simulink model "BWQWFPIDKZhShChU"  (Simulink 5.0)
settings: Solver=ode45  StartTime=0.0  StopTime=200  FixedStep=20  RelTol=1e-3
settings Model: LastModifiedBy=ThinkPad  RTWOptions="-aEnforceIntegerDowncast=1 -aExtMode=0 -aExtModeTesting=0 -aFoldNonRolledExpr=1 -aForceParamTrailComments=0 -aGenerateComments=1 -aGenerateReport=0 -aIgnoreCustomStorageClasses=1 -aIncDataTypeInIds=0 -aIncHierarchyInIds=0 -aInlineInvariantSignals=0 -aInlinedPrmAccess=\"Literals\" -aLocalBlockOutputs=1 -aLogVarNameModifier=\"rt_\" -aMaxRTWIdLen=31 -aPrefixModelToSubsysFcnNames=1 -aRTWVerbose=1 -aRollThreshold=5 -aShowEliminatedStatements=0"

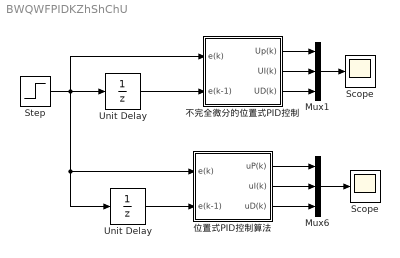
== system BWQWFPIDKZhShChU ==
  Mux1 : Mux  Inputs=3
  Mux6 : Mux  Inputs=3
  Scope : Scope
      settings: YMin=0  YMax=1.1  SaveName=BWQWFPID  DataFormat=Array  MaxDataPoints=500000
  "Scope " : Scope
      settings: YMin=0  YMax=2.5  SaveName=PID  DataFormat=Array  MaxDataPoints=500000
  "Step " : Step  Time=0  SampleTime=20
  Unit Delay : UnitDelay  SampleTime=20
  "Unit Delay " : UnitDelay  SampleTime=20
  不完全微分的位置式PID控制 : Subsystem
  "位置式PID控制算法 " : Subsystem
  wires:
  "Step "/1 -> Unit Delay/1, 不完全微分的位置式PID控制/1(e(k)), "Unit Delay "/1, "位置式PID控制算法 "/1(e(k))
  Unit Delay/1 -> 不完全微分的位置式PID控制/2(e(k-1))
  Mux1/1 -> Scope/1
  "Unit Delay "/1 -> "位置式PID控制算法 "/2(e(k-1))
  Mux6/1 -> "Scope "/1
  "位置式PID控制算法 "/1(uP(k)) -> Mux6/1
  "位置式PID控制算法 "/2(uI(k)) -> Mux6/2
  "位置式PID控制算法 "/3(uD(k)) -> Mux6/3
  不完全微分的位置式PID控制/2(UI(k)) -> Mux1/2
  不完全微分的位置式PID控制/3(UD(k)) -> Mux1/3
  不完全微分的位置式PID控制/1(Up(k)) -> Mux1/1

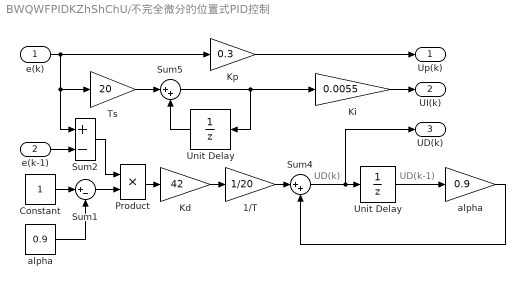
== system BWQWFPIDKZhShChU/不完全微分的位置式PID控制 ==
  note: UD(k)
  note: UD(k-1)
  e(k) : Inport
  e(k-1) : Inport  Port=2
  1/T : Gain  Gain=1/20  SaturateOnIntegerOverflow=on
  Constant : Constant
  Kd : Gain  Gain=42  SaturateOnIntegerOverflow=on
  Ki : Gain  Gain=0.0055  SaturateOnIntegerOverflow=on
  Kp : Gain  Gain=0.3  SaturateOnIntegerOverflow=on
  "Product " : Product  SaturateOnIntegerOverflow=on
  Sum1 : Sum  Inputs=|+-  SaturateOnIntegerOverflow=on
  Sum2 : Sum  Inputs=+-  SaturateOnIntegerOverflow=on
  Sum4 : Sum  Inputs=|++  SaturateOnIntegerOverflow=on
  Sum5 : Sum  Inputs=|++  SaturateOnIntegerOverflow=on
  Ts : Gain  Gain=20  SaturateOnIntegerOverflow=on
  Unit Delay : UnitDelay  SampleTime=20
  "Unit Delay " : UnitDelay  Orientation=left  SampleTime=20
  alpha : Constant  Value=0.9
  "alpha " : Gain  Gain=0.9  SaturateOnIntegerOverflow=on
  Up(k) : Outport
  UI(k) : Outport  Port=2
  UD(k) : Outport  Port=3
  wires:
  e(k)/1 -> Kp/1, Sum2/1, Ts/1
  Kp/1 -> Up(k)/1
  e(k-1)/1 -> Sum2/2
  Ki/1 -> UI(k)/1
  Constant/1 -> Sum1/1
  alpha/1 -> Sum1/2
  Sum2/1 -> "Product "/1
  Sum1/1 -> "Product "/2
  "Product "/1 -> Kd/1
  Kd/1 -> 1/T/1
  Sum4/1 -> Unit Delay/1, UD(k)/1
  Unit Delay/1 -> "alpha "/1
  "alpha "/1 -> Sum4/2
  1/T/1 -> Sum4/1
  Ts/1 -> Sum5/1
  Sum5/1 -> "Unit Delay "/1, Ki/1
  "Unit Delay "/1 -> Sum5/2

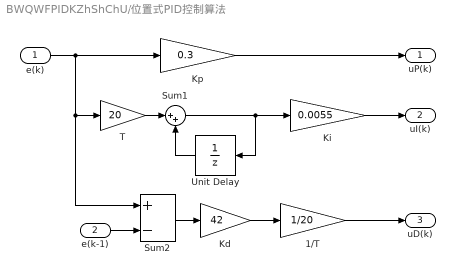
== system BWQWFPIDKZhShChU/位置式PID控制算法  ==
  e(k) : Inport
  e(k-1) : Inport  Port=2
  1/T : Gain  Gain=1/20  SaturateOnIntegerOverflow=on
  Kd : Gain  Gain=42  SaturateOnIntegerOverflow=on
  Ki : Gain  Gain=0.0055  SaturateOnIntegerOverflow=on
  Kp : Gain  Gain=0.3  SaturateOnIntegerOverflow=on
  Sum1 : Sum  Inputs=|++  SaturateOnIntegerOverflow=on
  Sum2 : Sum  Inputs=+-  SaturateOnIntegerOverflow=on
  T : Gain  Gain=20  SaturateOnIntegerOverflow=on
  "Unit Delay " : UnitDelay  Orientation=left  SampleTime=20
  uP(k) : Outport
  uI(k) : Outport  Port=2
  uD(k) : Outport  Port=3
  wires:
  Sum2/1 -> Kd/1
  e(k)/1 -> Kp/1, Sum2/1, T/1
  Kp/1 -> uP(k)/1
  Ki/1 -> uI(k)/1
  Kd/1 -> 1/T/1
  e(k-1)/1 -> Sum2/2
  1/T/1 -> uD(k)/1
  Sum1/1 -> "Unit Delay "/1, Ki/1
  "Unit Delay "/1 -> Sum1/2
  T/1 -> Sum1/1
